simulink model "Simulink_qu15_Barbier_Touboul"  (R2018b)
settings: Solver=FixedStepAuto  StartTime=0.0  StopTime=fin_15  FixedStep=dt_15  RelTol=1e-3
values from neighbouring files (symbols this model uses):
  A = [teta1;teta2]    [visualisation_trame.m]
  Kd_15 = 2*diag([1 1])    [visualisation_trame.m]
  Kp_15 = 110*diag([1 1])    [visualisation_trame.m]
undefined symbols (not defined in the file or in its folder): dyn, dyn2
settings Model: Creator=Claire  LastModifiedBy=Claire

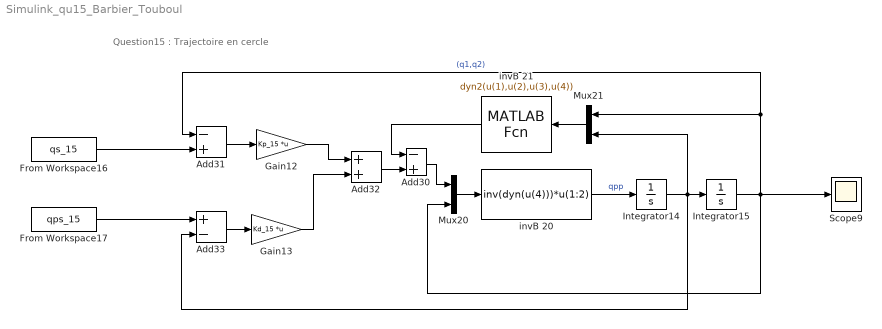
== system Simulink_qu15_Barbier_Touboul ==
  note: Question15 : Trajectoire en cercle
  Add30 : Sum  Inputs=-+
  Add31 : Sum  Inputs=-+
  Add32 : Sum
  Add33 : Sum  Inputs=+-
  From Workspace16 : FromWorkspace  VariableName=qs_15  SampleTime=0
  From Workspace17 : FromWorkspace  VariableName=qps_15  SampleTime=0
  Gain12 : Gain  Gain=Kp_15  Multiplication=Matrix(K*u)
  Gain13 : Gain  Gain=Kd_15  Multiplication=Matrix(K*u)
  Integrator14 : Integrator
  Integrator15 : Integrator  InitialCondition=[A(1,1) A(2,1)]
  Mux20 : Mux  Inputs=2
  Mux21 : Mux  Inputs=2
  Scope9 : Scope
  invB 20 : MATLABFcn  MATLABFcn=inv(dyn(u(4)))*u(1:2)  OutputDimensions=2
      mask Display: disp('inv(M)*Tau')
  invB 21 : MATLABFcn  MATLABFcn=dyn2(u(1),u(2),u(3),u(4))  OutputDimensions=2
      mask Display: disp('H(q,qp)')
  wires:
  From Workspace17/1 -> Add33/1
  From Workspace16/1 -> Add31/2
  Integrator15/1 -> Mux20/2, Scope9/1, Add31/1, Mux21/1  "(q1,q2)"
  Add31/1 -> Gain12/1
  Add30/1 -> Mux20/1
  Add33/1 -> Gain13/1
  Gain13/1 -> Add32/2
  Integrator14/1 -> Add33/2, Mux21/2, Integrator15/1
  Mux21/1 -> invB 21/1
  invB 21/1 -> Add30/1
  Add32/1 -> Add30/2
  Gain12/1 -> Add32/1
  Mux20/1 -> invB 20/1
  invB 20/1 -> Integrator14/1  "qpp"
